simulink model "HBA"  (R2023a)
settings: Solver=VariableStepAuto  StartTime=0.0  StopTime=10.0  RelTol=1e-3
undefined symbols (not defined in the file or in its folder): A_booster, A_master, Intial_vel, P_booster, RR
libraries: sdl_lib x9, nesl_utility x6, SignalEditorBlockLib x1
settings Model: Creator=Hossam_Selem  LastModifiedBy=Hossam_Selem

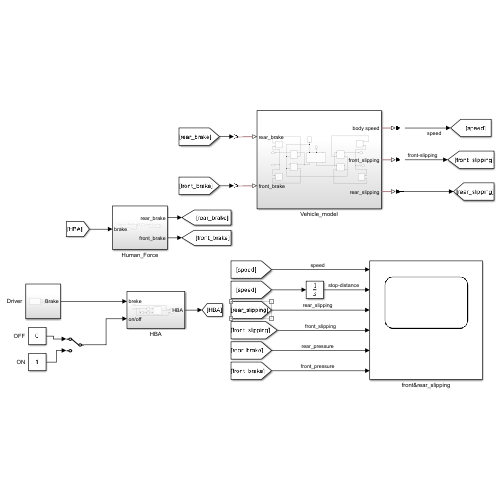
[thumbnail: Simulink's stored preview of the top-level diagram]
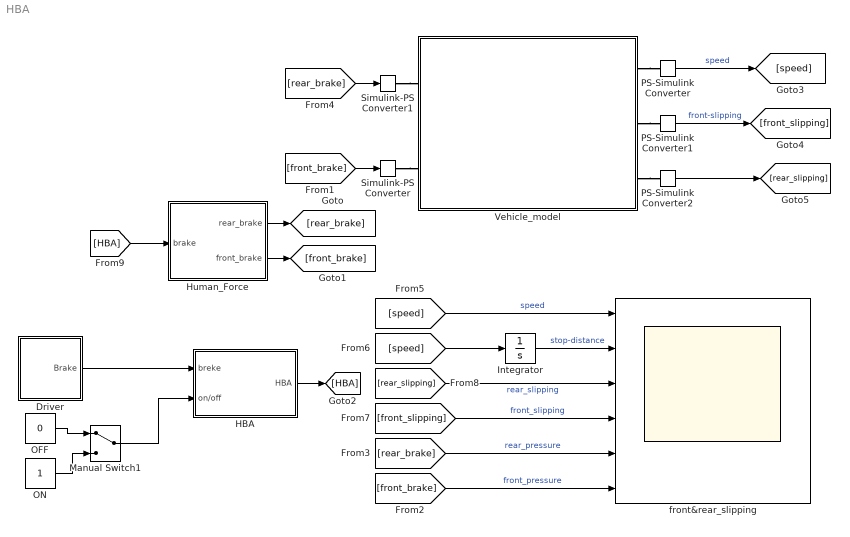
== system HBA ==
  Driver : Subsystem
  HBA : Subsystem
  Human_Force : Subsystem
  Integrator : Integrator
  Manual Switch1 : ManualSwitch
  OFF : Constant  Value=0
  ON : Constant
  PS-Simulink Converter : nesl_utility/PS-Simulink Converter  PhysicalDomain=network_engine_domain  SubClassName=ps_output  LeftPortType=input  RightPortType=output  PseudoPeriodic=off  Frequencies=[]  VectorFormat=inherit  Unit=m/s  AffineConversion=off
  PS-Simulink Converter1 : nesl_utility/PS-Simulink Converter  PhysicalDomain=network_engine_domain  SubClassName=ps_output  LeftPortType=input  RightPortType=output  PseudoPeriodic=off  Frequencies=[]  VectorFormat=1-D array  Unit=1  AffineConversion=off
  PS-Simulink Converter2 : nesl_utility/PS-Simulink Converter  PhysicalDomain=network_engine_domain  SubClassName=ps_output  LeftPortType=input  RightPortType=output  PseudoPeriodic=off  Frequencies=[]  VectorFormat=1-D array  Unit=1  AffineConversion=off
  Simulink-PS Converter : nesl_utility/Simulink-PS Converter  PhysicalDomain=network_engine_domain  SubClassName=ps_input  LeftPortType=input  RightPortType=output  PseudoPeriodic=off  Frequencies=[]  NoiseDistribution=none  NoiseParameters=[]  Unit=1  AffineConversion=off  FilteringAndDerivatives=provide  SimscapeFilterOrder=1  InputFilterTimeConstant=0.001  UdotUserProvided=0
  Simulink-PS Converter1 : nesl_utility/Simulink-PS Converter  PhysicalDomain=network_engine_domain  SubClassName=ps_input  LeftPortType=input  RightPortType=output  PseudoPeriodic=off  Frequencies=[]  NoiseDistribution=none  NoiseParameters=[]  Unit=1  AffineConversion=off  FilteringAndDerivatives=provide  SimscapeFilterOrder=1  InputFilterTimeConstant=0.001  UdotUserProvided=0
  Vehicle_model : Subsystem
  front&rear_slipping : Scope  NumInputPorts=6
  wires:
  Human_Force/1(rear_brake) -> [rear_brake]
  Human_Force/2(front_brake) -> [front_brake]
  PS-Simulink Converter/1 -> [speed]  "speed"
  [rear_brake] -> Simulink-PS Converter1/1
  [front_brake] -> Simulink-PS Converter/1
  PS-Simulink Converter1/1 -> [front_slipping]  "front-slipping"
  PS-Simulink Converter2/1 -> [rear_slipping]
  [rear_slipping] -> front&rear_slipping/3  "rear_slipping"
  [front_slipping] -> front&rear_slipping/4  "front_slipping"
  [speed] -> Integrator/1
  [speed] -> front&rear_slipping/1  "speed"
  [rear_brake] -> front&rear_slipping/5  "rear_pressure"
  [front_brake] -> front&rear_slipping/6  "front_pressure"
  Integrator/1 -> front&rear_slipping/2  "stop-distance"
  [HBA] -> Human_Force/1(brake)
  HBA/1(HBA) -> [HBA]
  Driver/1(Brake) -> HBA/1(breke)
  Manual Switch1/1 -> HBA/2(on/off)
  ON/1 -> Manual Switch1/2
  OFF/1 -> Manual Switch1/1
  connections:
  Vehicle_model/RConn2 -- PS-Simulink Converter1/LConn1
  Simulink-PS Converter1/RConn1 -- Vehicle_model/LConn1
  Vehicle_model/RConn1 -- PS-Simulink Converter/LConn1
  Vehicle_model/RConn3 -- PS-Simulink Converter2/LConn1
  Simulink-PS Converter/RConn1 -- Vehicle_model/LConn2

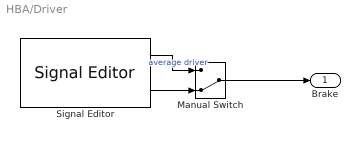
== system HBA/Driver ==
  Manual Switch : ManualSwitch  CurrentSetting=0
  Signal Editor : SignalEditorBlockLib/Signal Editor  FileName=untitled.mat  ActiveScenario=Scenario  ActiveSignal=Signal 1  IsBus=off  OutputBusObjectStr=Bus: BusObject  SampleTime=0  Interpolate=off  ZeroCross=off  OutputAfterFinalValue=Setting to zero  Unit=inherit  PreserveSignalName=on  ApplySigPropsToAllScenarios=on
  Brake : Outport
  wires:
  Signal Editor/2 -> Manual Switch/2
  Manual Switch/1 -> Brake/1
  Signal Editor/1 -> Manual Switch/1  "average driver"

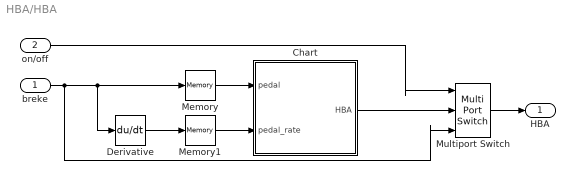
== system HBA/HBA ==
  breke : Inport
  on/off : Inport  Port=2
  Chart : Stateflow chart  TreatAsAtomicUnit=on
  Derivative : Derivative
  Memory : Memory
  Memory1 : Memory
  Multiport Switch : MultiPortSwitch  DataPortOrder=Specify indices  Inputs=2  DataPortIndices={1,0}  SaturateOnIntegerOverflow=off  InputSameDT=off
  HBA : Outport
  wires:
  breke/1 -> Multiport Switch/3, Derivative/1, Memory/1
  Memory1/1 -> Chart/2(pedal_rate)
  Memory/1 -> Chart/1(pedal)
  Chart/1(HBA) -> Multiport Switch/2
  Multiport Switch/1 -> HBA/1
  Derivative/1 -> Memory1/1
  on/off/1 -> Multiport Switch/1

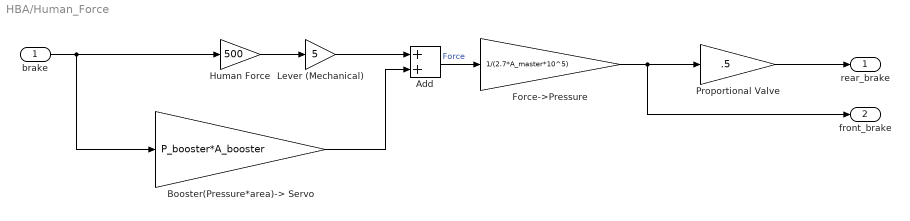
== system HBA/Human_Force ==
  brake : Inport
  Add : Sum
  Booster(Pressure*area)-> Servo : Gain  Gain=P_booster*A_booster
  Force->Pressure : Gain  Gain=1/(2.7*A_master*10^5)
  Human Force : Gain  Gain=500
  Lever (Mechanical) : Gain  Gain=5
  Proportional Valve : Gain  Gain=.5
  rear_brake : Outport
  front_brake : Outport  Port=2
  wires:
  Proportional Valve/1 -> rear_brake/1
  Lever (Mechanical)/1 -> Add/1
  brake/1 -> Booster(Pressure*area)-> Servo/1, Human Force/1
  Human Force/1 -> Lever (Mechanical)/1
  Add/1 -> Force->Pressure/1  "Force"
  Booster(Pressure*area)-> Servo/1 -> Add/2
  Force->Pressure/1 -> Proportional Valve/1, front_brake/1

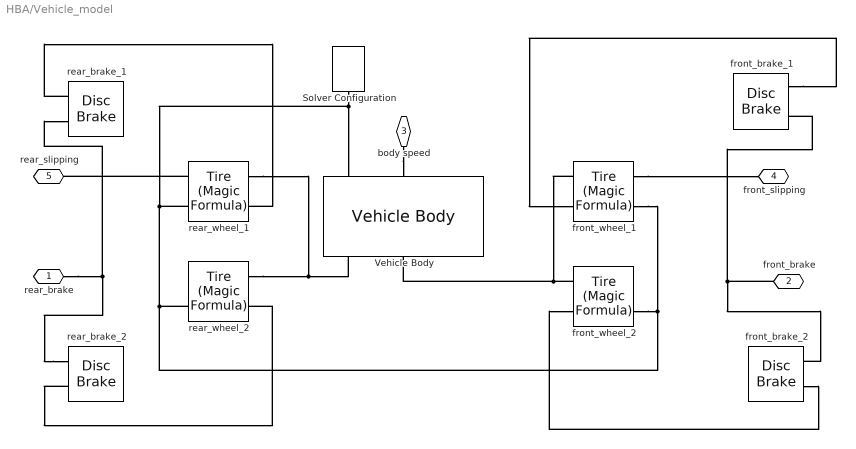
== system HBA/Vehicle_model ==
  Solver Configuration : nesl_utility/Solver Configuration  PhysicalDomain=network_engine_domain  SubClassName=solver  LeftPortType=input  RightPortType=generic  Tones=[]  Harmonics=[]  SimulateNoise=off  Profile=off  UseLocalSampling=off  EnableSwitchedLinearOptims=on  FrequencyDomain=off  UseCCode=off  RelTol=0.001  AbsTol=0.001  MinStep=1e-09  ToWorkspace=off  RevertToSquareIcSolve=off  NumHomotopyIterations=100  PhasorMode=off  PhasorModeNumHarmonics=1  ConsistencySolver=NEWTON_XTOL_AFTER_FTOL  IndexReductionMethod=DerivativeReplacement  DoDC=off  ResidualTolerance=1e-09  ConsistencyTolSource=GLOBAL  ConsistencyAbsTol=0.001  ConsistencyRelTol=0.001  ConsistencyTolFactor=0.001  UseLocalSolver=off  LocalSolverChoice=NE_BACKWARD_EULER_ADVANCER  ResolveIndetEquations=on  FunctionEvalNumThread=1  LocalSolverSampleTime=0.001  DoFixedCost=off  MaxNonlinIter=3  MaxModeIter=2  ComputeImpulses=off  ImpulseIterations=2  LinearAlgebra=auto  LinearAlgebraNumThread=0  EquationFormulation=NE_TIME_EF  DelaysMemoryBudget=1024  AutomaticFiltering=on  FilteringTimeConstant=0.001  PartitionStorageMethod=AS_NEEDED  PartitionMemoryBudget=1024  PartitionMethod=ROBUST
  Vehicle Body : sdl_lib/Tires & Vehicles/Vehicle Body  mass=M_body kg  n_w=2  x_f=CG_Front m  x_r=CG_Rear m  y_c=CG_height m  mass_var=simscape.enum.onoff.off  g=9.81 m/s^2  liftoff_warning=simscape.enum.onoff.off  area=Front_Area m^2  Cd=Drag_Cof  rho=1.18 kg/m^3  model_pitch=simscape.enum.onoff.off  inertia=2500 kg*m^2  suspension_model=sdl.enum.linearTLU.linear  k_f=25000 N/m  b_f=2000 N*s/m  k_r=20000 N/m  b_r=1800 N*s/m  k_f_TLU=[-2000, -1000, 0, 1000, 2000] N  x_f_TLU=[-.4, -.2, 0, .2, .4] m  b_f_TLU=[-200, -100, 0, 100, 200] N  v_f_TLU=[-4, -2, 0, 2, 4] m/s  k_r_TLU=[-2000, -1000, 0, 1000, 2000] N  x_r_TLU=[-.4, -.2, 0, .2, .4] m  b_r_TLU=[-200, -100, 0, 100, 200] N  v_r_TLU=[-4, -2, 0, 2, 4] m/s  interp_method=simscape.enum.interpolation.linear  extrap_method=simscape.enum.extrapolation.linear  model_hardstop=simscape.enum.onoff.off  upper_bound_f=.25 m  lower_bound_f=-.25 m  stop_k_f=1e6 N/m  stop_b_f=150 N*s/m  upper_bound_r=.25 m  lower_bound_r=-.25 m  stop_k_r=1e6 N/m  stop_b_r=150 N*s/m  initial_pitch=0 rad  initial_pitch_rate=0 rad/s  v_specify=on  v_priority=High  v=Intial_vel m/s  v_nominal_specify=off  v_nominal_unit=kph  v_nominal_value=0
  front_brake_1 : sdl_lib/Brakes & Detents/Rotational/Disc Brake  r_mean=MPR mm  bore=CB mm  n_pads=2  thermal_port=simscape.enum.thermaleffects.omit  mu_static=SFC  mu_coulomb=CFC  temperature_TLU=[280, 300, 320] K  mu_static_TLU=[.9, .8, .7]  mu_coulomb_TLU=[.8, .7, .6]  brkwy_vel=BFV rad/s  visc_coef=VFC N*m*s/rad  enable_faults=simscape.enum.onoff.off  faulted_pressure=0 bar  external_fault=simscape.enum.onoff.off  temporal_fault=simscape.enum.onoff.off  fault_time=5 s  report_fault=simscape.enum.assert.action.none  thermal_mass=50 kJ/K  temperature_specify=off  temperature_priority=High  temperature=300 K  temperature_nominal_specify=off  temperature_nominal_unit=K  temperature_nominal_value=1
  front_brake_2 : sdl_lib/Brakes & Detents/Rotational/Disc Brake  r_mean=MPR mm  bore=CB mm  n_pads=2  thermal_port=simscape.enum.thermaleffects.omit  mu_static=SFC  mu_coulomb=CFC  temperature_TLU=[280, 300, 320] K  mu_static_TLU=[.9, .8, .7]  mu_coulomb_TLU=[.8, .7, .6]  brkwy_vel=BFV rad/s  visc_coef=VFC N*m*s/rad  enable_faults=simscape.enum.onoff.off  faulted_pressure=0 bar  external_fault=simscape.enum.onoff.off  temporal_fault=simscape.enum.onoff.off  fault_time=5 s  report_fault=simscape.enum.assert.action.none  thermal_mass=50 kJ/K  temperature_specify=off  temperature_priority=High  temperature=300 K  temperature_nominal_specify=off  temperature_nominal_unit=K  temperature_nominal_value=1
  front_wheel_1 : sdl_lib/Tires & Vehicles/Tire (Magic Formula)  parameterization=sdl.enum.magic_tire_model.peak  F_z1=RVL N  F_x1=PLF N  kappa1=Slip  B_m=10  C_m=1.9  D_m=1  E_m=0.97  fz0=4000 N  p_Cx=1.685  p_Dx=[1.21, -.037]  p_Ex=[.344, .095, -.02, 0]  p_Kx=[21.51, -.163, .245]  p_Hx=[-.002, .002]  p_Vx=[0, 0]  rolling_radius_model=sdl.enum.RollingRadiusParameterization.Constant  r_e=RR m  r_0=0.3 m  breff=8.39  dreff=0.26  freff=0.074  q_re0=0.99  q_v1=0.008  longvl=17 m/s  cz=5e5 N/m  model_resistance=false  resistance_model=sdl.enum.rollingResistanceParameterization.constant  coeff=0.015  p_tire=250e3 Pa  alpha=-0.003  beta=0.97  coeff_a=84e-4  coeff_b=6.2e-4 s/m  coeff_c=1.6e-4 s^2/m^2  p_tire0=240e3 Pa  fz0_resistance=4000 N  vH0=16 m/s  q_Sy=[.0082, 0, .0014, .001, 0, 0, 1.08, -.5]  v_thr=0.001 m/s  enable_scaling_coefficients=false  lfzO=1  lcx=1  lmux=1  lex=1  lkx=1  lhx=1  lvx=1  lmy=1  model_compliance=sdl.enum.compliance.off  stiffness=1e6 N/m  damping=1000 N*s/m  model_inertia=sdl.enum.model_inertia.on  inertia=TI kg*m^2  initial_velocity=(Intial_vel/RR) rad/s  vxlow=1 m/s  v_tr_thr=0.1 m/s  kpumin=-1.5  kpumax=1.5
  front_wheel_2 : sdl_lib/Tires & Vehicles/Tire (Magic Formula)  parameterization=sdl.enum.magic_tire_model.peak  F_z1=RVL N  F_x1=PLF N  kappa1=Slip  B_m=10  C_m=1.9  D_m=1  E_m=0.97  fz0=4000 N  p_Cx=1.685  p_Dx=[1.21, -.037]  p_Ex=[.344, .095, -.02, 0]  p_Kx=[21.51, -.163, .245]  p_Hx=[-.002, .002]  p_Vx=[0, 0]  rolling_radius_model=sdl.enum.RollingRadiusParameterization.Constant  r_e=RR m  r_0=0.3 m  breff=8.39  dreff=0.26  freff=0.074  q_re0=0.99  q_v1=0.008  longvl=17 m/s  cz=5e5 N/m  model_resistance=false  resistance_model=sdl.enum.rollingResistanceParameterization.constant  coeff=0.015  p_tire=250e3 Pa  alpha=-0.003  beta=0.97  coeff_a=84e-4  coeff_b=6.2e-4 s/m  coeff_c=1.6e-4 s^2/m^2  p_tire0=240e3 Pa  fz0_resistance=4000 N  vH0=16 m/s  q_Sy=[.0082, 0, .0014, .001, 0, 0, 1.08, -.5]  v_thr=0.001 m/s  enable_scaling_coefficients=false  lfzO=1  lcx=1  lmux=1  lex=1  lkx=1  lhx=1  lvx=1  lmy=1  model_compliance=sdl.enum.compliance.off  stiffness=1e6 N/m  damping=1000 N*s/m  model_inertia=sdl.enum.model_inertia.on  inertia=TI kg*m^2  initial_velocity=(Intial_vel/RR) rad/s  vxlow=1 m/s  v_tr_thr=0.1 m/s  kpumin=-1.5  kpumax=1.5
  rear_brake_1 : sdl_lib/Brakes & Detents/Rotational/Disc Brake  r_mean=MPR mm  bore=CB mm  n_pads=2  thermal_port=simscape.enum.thermaleffects.omit  mu_static=SFC  mu_coulomb=CFC  temperature_TLU=[280, 300, 320] K  mu_static_TLU=[.9, .8, .7]  mu_coulomb_TLU=[.8, .7, .6]  brkwy_vel=BFV rad/s  visc_coef=VFC N*m*s/rad  enable_faults=simscape.enum.onoff.off  faulted_pressure=0 bar  external_fault=simscape.enum.onoff.off  temporal_fault=simscape.enum.onoff.off  fault_time=5 s  report_fault=simscape.enum.assert.action.none  thermal_mass=50 kJ/K  temperature_specify=off  temperature_priority=High  temperature=300 K  temperature_nominal_specify=off  temperature_nominal_unit=K  temperature_nominal_value=1
  rear_brake_2 : sdl_lib/Brakes & Detents/Rotational/Disc Brake  r_mean=MPR mm  bore=CB mm  n_pads=2  thermal_port=simscape.enum.thermaleffects.omit  mu_static=SFC  mu_coulomb=CFC  temperature_TLU=[280, 300, 320] K  mu_static_TLU=[.9, .8, .7]  mu_coulomb_TLU=[.8, .7, .6]  brkwy_vel=BFV rad/s  visc_coef=VFC N*m*s/rad  enable_faults=simscape.enum.onoff.off  faulted_pressure=0 bar  external_fault=simscape.enum.onoff.off  temporal_fault=simscape.enum.onoff.off  fault_time=5 s  report_fault=simscape.enum.assert.action.none  thermal_mass=50 kJ/K  temperature_specify=off  temperature_priority=High  temperature=300 K  temperature_nominal_specify=off  temperature_nominal_unit=K  temperature_nominal_value=1
  rear_wheel_1 : sdl_lib/Tires & Vehicles/Tire (Magic Formula)  parameterization=sdl.enum.magic_tire_model.peak  F_z1=RVL N  F_x1=PLF N  kappa1=Slip  B_m=10  C_m=1.9  D_m=1  E_m=0.97  fz0=4000 N  p_Cx=1.685  p_Dx=[1.21, -.037]  p_Ex=[.344, .095, -.02, 0]  p_Kx=[21.51, -.163, .245]  p_Hx=[-.002, .002]  p_Vx=[0, 0]  rolling_radius_model=sdl.enum.RollingRadiusParameterization.Constant  r_e=RR m  r_0=0.3 m  breff=8.39  dreff=0.26  freff=0.074  q_re0=0.99  q_v1=0.008  longvl=17 m/s  cz=5e5 N/m  model_resistance=false  resistance_model=sdl.enum.rollingResistanceParameterization.constant  coeff=0.015  p_tire=250e3 Pa  alpha=-0.003  beta=0.97  coeff_a=84e-4  coeff_b=6.2e-4 s/m  coeff_c=1.6e-4 s^2/m^2  p_tire0=240e3 Pa  fz0_resistance=4000 N  vH0=16 m/s  q_Sy=[.0082, 0, .0014, .001, 0, 0, 1.08, -.5]  v_thr=0.001 m/s  enable_scaling_coefficients=false  lfzO=1  lcx=1  lmux=1  lex=1  lkx=1  lhx=1  lvx=1  lmy=1  model_compliance=sdl.enum.compliance.off  stiffness=1e6 N/m  damping=1000 N*s/m  model_inertia=sdl.enum.model_inertia.on  inertia=TI kg*m^2  initial_velocity=(Intial_vel/RR) rad/s  vxlow=1 m/s  v_tr_thr=0.1 m/s  kpumin=-1.5  kpumax=1.5
  rear_wheel_2 : sdl_lib/Tires & Vehicles/Tire (Magic Formula)  parameterization=sdl.enum.magic_tire_model.peak  F_z1=RVL N  F_x1=PLF N  kappa1=Slip  B_m=10  C_m=1.9  D_m=1  E_m=0.97  fz0=4000 N  p_Cx=1.685  p_Dx=[1.21, -.037]  p_Ex=[.344, .095, -.02, 0]  p_Kx=[21.51, -.163, .245]  p_Hx=[-.002, .002]  p_Vx=[0, 0]  rolling_radius_model=sdl.enum.RollingRadiusParameterization.Constant  r_e=RR m  r_0=0.3 m  breff=8.39  dreff=0.26  freff=0.074  q_re0=0.99  q_v1=0.008  longvl=17 m/s  cz=5e5 N/m  model_resistance=false  resistance_model=sdl.enum.rollingResistanceParameterization.constant  coeff=0.015  p_tire=250e3 Pa  alpha=-0.003  beta=0.97  coeff_a=84e-4  coeff_b=6.2e-4 s/m  coeff_c=1.6e-4 s^2/m^2  p_tire0=240e3 Pa  fz0_resistance=4000 N  vH0=16 m/s  q_Sy=[.0082, 0, .0014, .001, 0, 0, 1.08, -.5]  v_thr=0.001 m/s  enable_scaling_coefficients=false  lfzO=1  lcx=1  lmux=1  lex=1  lkx=1  lhx=1  lvx=1  lmy=1  model_compliance=sdl.enum.compliance.off  stiffness=1e6 N/m  damping=1000 N*s/m  model_inertia=sdl.enum.model_inertia.on  inertia=TI kg*m^2  initial_velocity=(Intial_vel/RR) rad/s  vxlow=1 m/s  v_tr_thr=0.1 m/s  kpumin=-1.5  kpumax=1.5
  rear_brake : PMIOPort  Side=Left
  front_brake : PMIOPort  Port=2  Side=Left
  body speed : PMIOPort  Port=3  Side=Right
  front_slipping : PMIOPort  Port=4  Side=Right
  rear_slipping : PMIOPort  Port=5  Side=Right
  connections:
  rear_wheel_1/RConn1 -- rear_slipping/RConn1
  rear_brake_1/LConn2 -- rear_wheel_1/LConn2
  rear_brake_2/LConn1 -- rear_brake_1/LConn1 -- rear_brake/RConn1
  rear_brake_2/LConn2 -- rear_wheel_2/LConn2
  Vehicle Body/RConn2 -- front_wheel_2/LConn1 -- front_wheel_1/LConn1
  body speed/RConn1 -- Vehicle Body/LConn2
  front_wheel_1/RConn1 -- front_slipping/RConn1
  rear_wheel_2/RConn2 -- front_wheel_2/RConn2 -- front_wheel_1/RConn2 -- Solver Configuration/RConn1 -- Vehicle Body/LConn1 -- rear_wheel_1/RConn2
  front_brake_2/LConn2 -- front_wheel_2/LConn2
  Vehicle Body/RConn1 -- rear_wheel_2/LConn1 -- rear_wheel_1/LConn1
  front_brake_1/LConn2 -- front_wheel_1/LConn2
  front_brake_2/LConn1 -- front_brake_1/LConn1 -- front_brake/RConn1

== stateflow chart HBA/Chart ==
  state normal
    HBA=pedal
  state active
    HBA=1
  (default) -> normal
  normal -> active : [pedal_rate<0.1]
  active -> normal : [pedal_rate>0.2]
  data: pedal input; HBA output; pedal_rate input
